simulink model "Refined_Model_43_Elec5_ch"  (R2020b)
settings: Solver=VariableStepAuto  StartTime=0.0  StopTime=16000  RelTol=1e-3
values from neighbouring files (symbols this model uses):
  Cx = VehicleDefine(7,3)    [BEV_Script_GPS.m]    (also in ICEBEV_Script_GPS.m; ICE_Script_GPS.m)
  Dist = [1:length(FMSP1)]    [BEV_Script_GPS.m]    (also in ICEBEV_Script_GPS.m; ICE_Script_GPS.m)
  DynRolRad = VehicleDefine(5,3)    [BEV_Script_GPS.m]    (also in ICEBEV_Script_GPS.m; ICE_Script_GPS.m)
  Fr = VehicleDefine(13,3)    [BEV_Script_GPS.m]    (also in ICEBEV_Script_GPS.m; ICE_Script_GPS.m)
  g = VehicleDefine(14,3)    [BEV_Script_GPS.m]    (also in ICEBEV_Script_GPS.m; ICE_Script_GPS.m)
  IntpSlope = round(IntpSlope,1)    [BEV_Script_GPS.m]    (also in ICEBEV_Script_GPS.m; ICE_Script_GPS.m)
  MaxAcc = 1    [BEV_Script_GPS.m]    (also in ICEBEV_Script_GPS.m; ICE_Script_GPS.m)
  MaxDec = 1    [BEV_Script_GPS.m]    (also in ICEBEV_Script_GPS.m; ICE_Script_GPS.m)
  MaxSpeedProfile = repelem(SegSPLatinmps,SegLeninm)    [BEV_Script_GPS.m]    (also in ICEBEV_Script_GPS.m; ICE_Script_GPS.m)
  Mtot = Mv+Me+Mt    [BEV_Script_GPS.m]    (also in ICEBEV_Script_GPS.m; ICE_Script_GPS.m)
  rho = VehicleDefine(6,3)    [BEV_Script_GPS.m]    (also in ICEBEV_Script_GPS.m; ICE_Script_GPS.m)
  s = divisors(length(MaxSpeedProfile))    [BEV_Script_GPS.m]    (also in ICEBEV_Script_GPS.m; ICE_Script_GPS.m; interparc.m = totalsplinelength*t)
  SegSPLatinmps = (sqrt(aMaxLat*g*CurRadinm))    [BEV_Script_GPS.m]    (also in ICEBEV_Script_GPS.m; ICE_Script_GPS.m)
  Stoptimes = readmatrix('GPS Routes and OC\Brno - Vienna - OC_description.xlsx','Sheet','Stop')    [BEV_Script_GPS.m]    (also in ICEBEV_Script_GPS.m = readmatrix('GPS Routes and OC\Turin - Lyon - OC_description.; ICE_Script_GPS.m = readmatrix('GPS Routes and OC\Dusseldorf - Cologne - OC_desc)
  Sx = VehicleDefine(8,3)    [BEV_Script_GPS.m]    (also in ICEBEV_Script_GPS.m; ICE_Script_GPS.m)
  W_mmax = VehicleDefine(26,3)    [BEV_Script_GPS.m]    (also in ICEBEV_Script_GPS.m = Etr(1,3))
undefined symbols (not defined in the file or in its folder): CovDist, G1Inprpm, Ion, Lithium, SegNo
libraries: fl_lib x8, nesl_utility x4, ee_lib x3, powerlib x2, electricdrivelib x1, sdl_lib x1, autolibshared x1
settings Model: Creator=Kshitij  LastModifiedBy=Kshitij
settings SolverCC: MaxConsecutiveMinStep=100000  ZeroCrossAlgorithm=Adaptive
settings DebuggingCC: IgnoredZcDiagnostic=none

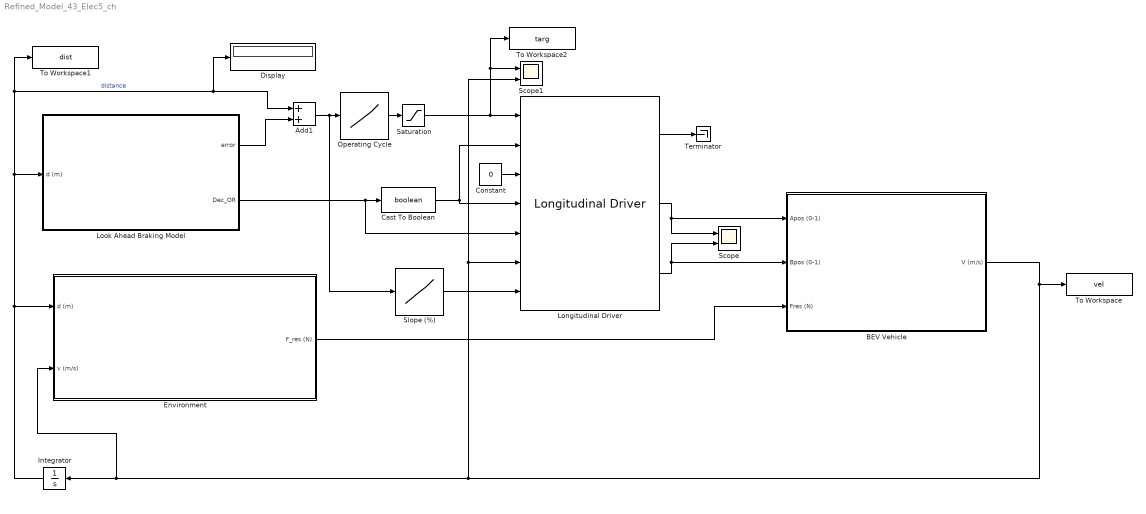
== system Refined_Model_43_Elec5_ch ==
  Add1 : Sum
  BEV Vehicle : Subsystem
  Cast To Boolean : DataTypeConversion  OutDataTypeStr=boolean
  Constant : Constant  Value=0
  Display : Display
  Environment : Subsystem
  Integrator : Integrator
  Longitudinal Driver : autolibshared/Longitudinal Driver  extAccelOvr=on  extDecelOvr=on  extAccelHld=off  extDecelHld=off  extAccelZero=off  extDecelZero=off  cntrlType=PI  shftType=None  velUnits=m/s  gearOut=off  Kp=200  Ki=150  Kff=0  Kg=0  VehVelVec=[0 100]  KffVec=[.1 .1]  KpVec=[10 10]  KiVec=[5 5]  KgVec=[0 0]  m=1500  Kpt=3000  tau=.1  L=2  aR=200  bR=2.5  cR=.5  g=9.81  vnom=100  Kaw=0  tauerr=0  tauPt=2  GearInit=0  tShift=.1  pdlVec=[0.1 0.4 0.5 0.9]  upShftTbl=[-1 12.9375 26.4375 39.9375 51.18749999999999 62.4375 72.84375 83.25;-1 16.3125 29.8125 43.3125 54.5624 65.8125 76.78125 87.75;-1 19.6875 33.1875 46.68749999999999 57.9375 69.1875 80.71875 92.25;-1 33 52.5 77.25 100.5 138.75 161.875 185]  dwnShftTbl=[1 9.5625 23.0625 36.5625 47.8125 59.0625 68.90625 78.75;1 12.9375 26.4375 39.9375 51.18749999999999 62.4375 72.84375 83.25;1 16.3125 29.8125 43.3125 54.562499 65.8125 76.78125 87.75;1 19.6875 33.1875 46.68749999999999 57.9375 69.1875 80.71875 92.25]  tClutch=.5  tRev=.5  tPark=120  aMode=1  UpGearVec="[0  1  2  3  4  5  6  7]"  DownGearVec="[1  2  3  4  5  6  7  8]"
      settings: SourceProductBaseCode=PW,DR,MT,UV,VE
  Look Ahead Braking Model : Subsystem
  Operating Cycle : Lookup_n-D  NumberOfTableDimensions=1  BreakpointsForDimension1=Dist  BreakpointsForDimension2=G1Inprpm  Table=MaxSpeedProfile  InterpMethod=Linear Lagrange  InternalRulePriority=Speed  RndMeth=Simplest  InputSameDT=on
  Saturation : Saturate  UpperLimit=inf  LowerLimit=0
  Scope : Scope  NumInputPorts=2
  Scope1 : Scope  NumInputPorts=2
  Slope (%) : Lookup_n-D  NumberOfTableDimensions=1  BreakpointsForDimension1=Dist  Table=IntpSlope  InternalRulePriority=Speed  RndMeth=Simplest  InputSameDT=on
  Terminator : Terminator
  To Workspace : ToWorkspace  VariableName=vel  SaveFormat=Timeseries  SampleTime=-1
  To Workspace1 : ToWorkspace  VariableName=dist  SaveFormat=Timeseries  SampleTime=-1
  To Workspace2 : ToWorkspace  VariableName=targ  SaveFormat=Timeseries  SampleTime=-1
  wires:
  Longitudinal Driver/2 -> Scope/1, BEV Vehicle/1(Apos (0-1))
  Integrator/1 -> To Workspace1/1, Add1/1, Display/1, Look Ahead Braking Model/1(d (m)), Environment/1(d (m))  "distance"
  Slope (%)/1 -> Longitudinal Driver/7
  Operating Cycle/1 -> Saturation/1
  Longitudinal Driver/1 -> Terminator/1
  Look Ahead Braking Model/2(Dec_OR) -> Longitudinal Driver/5, Cast To Boolean/1
  Cast To Boolean/1 -> Longitudinal Driver/4, Longitudinal Driver/2
  Add1/1 -> Slope (%)/1, Operating Cycle/1
  Look Ahead Braking Model/1(error) -> Add1/2
  BEV Vehicle/1(V (m/s)) -> To Workspace/1, Scope1/2, Longitudinal Driver/6, Environment/2(v (m/s)), Integrator/1
  Longitudinal Driver/3 -> BEV Vehicle/2(Bpos (0-1)), Scope/2
  Environment/1(F_res (N)) -> BEV Vehicle/3(Fres (N))
  Saturation/1 -> To Workspace2/1, Scope1/1, Longitudinal Driver/1
  Constant/1 -> Longitudinal Driver/3

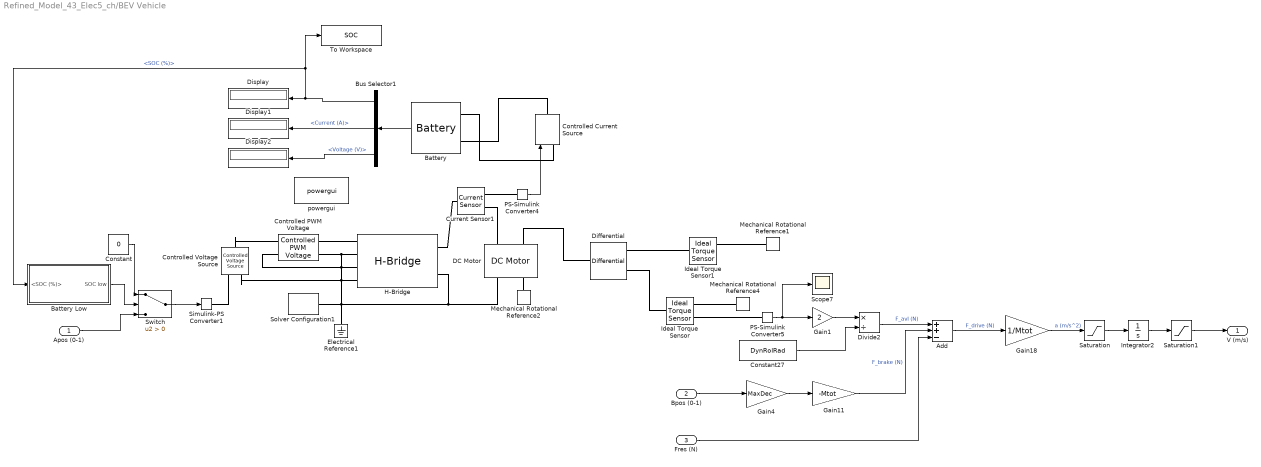
== system Refined_Model_43_Elec5_ch/BEV Vehicle ==
  Apos (0-1) : Inport
  Bpos (0-1) : Inport  Port=2
  Fres (N) : Inport  Port=3
  Add : Sum  Inputs=++-
  Battery : electricdrivelib/Extra Sources/Battery  BatType=Lithium-Ion  ShowTempParam=off  ThermalPreset=no  ShowAgeParam=off  NomV=V  NomQ=C_cap  SOC=100  Batt_Tr=15  PresetModel=on  MaxQ=470  MinV=562.5  FullV=872.9904  Dis_rate=204.3478  R=0.015957  Normal_OP=425.0435  expZone="[810.2894       23.0913]"  current=[6.5 13 32.5]  Units=Time  Tci=20  NomT=20  T2=-30  MaxQ2=4.8  FullV2=7.1  Normal_OP2=5.655  expZone2="[6.58           1]"  Rca=0.6  ti=2000  Dp=0  Neq0=0  Tsim=1e6  Ta1=25  Qeol=5.4*0.9  Reol=0.013333*1.2  Char_age=[2.3478, 3]  Dis_age=[2.3478, 10]  N1=1500  N2=10500  N3=1000  N4=1400  Ta2=45  N5=950
  Battery Low : Subsystem
  Bus Selector1 : BusSelector  OutputSignals=SOC (%),Current (A),Voltage (V)
  Constant : Constant  Value=0
  Constant27 : Constant  Value=DynRolRad
  Controlled Current Source : powerlib/Electrical Sources/Controlled Current Source  Initialize=on  Source_Type=DC  Amplitude=0  Phase=0  Frequency=0  Measurements=None
  Controlled PWM Voltage : ee_lib/Integrated Circuits/Controlled PWM Voltage  F=1000 Hz  TD=0 s  pulse_width_offset=0 s  pulse_min=0 s  Vmin=0 V  Vmax=2.5 V  Vm=V V  pwm_or_av=2  event_type=1  sample_time=1e-6 s  u_min=0  u_max=1
  Controlled Voltage Source : fl_lib/Electrical/Electrical Sources/Controlled Voltage Source
  Current Sensor1 : fl_lib/Electrical/Electrical Sensors/Current Sensor
  DC Motor : ee_lib/Electromechanical/Brushed Motors/DC Motor  field_option=ee.enum.field_option.pm  Rf=100 Ohm  Lf=1 H  Laf=0.15 H  If0=0 A  parameterization=ee.enum.dcparam_option.load_speed  Ra=3.9 Ohm  La=12e-6 H  emf_or_torque=ee.enum.emf_or_torque.kv  Kv=0.072e-3 V/rpm  Ki=6.876e-4 N*m/A  T_stall=0.24e-3 N*m  w_max=W_mmax rpm  w_rated=W_mmax-200 rpm  P_rated=P_mmax kW  V_rated=V V  J=0.01 g*cm^2  lam_param=ee.enum.lam_param.damping  lam=0 N*m/(rad/s)  i_noload=0 A  V_i_noload=1.5 V  speed0=0 rpm  enable_fault_armature=ee.enum.faults.faultEnable.no  rev_faulted=1 / 3  G_faulted_armature=1e-5 S  fault_trigger_armature=ee.enum.faults.faultTrigger.temporal  t_fault_armature=1 s  max_permissible_current_armature=inf A  t_fail_on_current_armature=1 s  enable_fault_field=ee.enum.faults.faultEnable.no  G_faulted_field=1e-5 S  fault_trigger_field=ee.enum.faults.faultTrigger.temporal  t_fault_field=1 s  max_permissible_current_field=inf A  t_fail_on_current_field=1 s  fault_action=ee.enum.faults.faultAction.none  alpha=3.93e-3 1/K  Tmeas=25 degC  thermal_mass=100 J/K  initial_temperature=25 degC
  Differential : sdl_lib/Gears/Differential  driveshaft_location=sdl.enum.differential_orientation.right  cd_ratio=FDR  friction_model=sdl.enum.gear_friction.none  mu_visc=[0, 0] N*m/(rad/s)  efficiency=[.85, .92]  temperature_TLU=[280, 300, 320] K  efficiency_ss_TLU=[.95, .9, .85]  efficiency_cd_TLU=[.95, .9, .85]  pwr_thr=[.001, .001] W  thermal_mass=50 J/K  T_init=300 K  model_inertia=simscape.enum.onoff.off  carrier_inertia=0.001 kg*m^2  planet_inertia=0.001 kg*m^2
      settings: SourceProductBaseCode=LD
  Display : Display
  Display1 : Display
  Display2 : Display
  Divide2 : Product  Inputs=*/
  Electrical Reference1 : fl_lib/Electrical/Electrical Elements/Electrical Reference
  Gain1 : Gain  Gain=2
  Gain11 : Gain  Gain=-Mtot
  Gain18 : Gain  Gain=1/Mtot
  Gain4 : Gain  Gain=MaxDec
  H-Bridge : ee_lib/Semiconductors & Converters/Converters/H-Bridge  supply_ports=ee.enum.supply_ports.hidesupply  Venable=2.5 V  Vmax=5.0 V  Vreverse=2.5 V  Vbrake=2.5 V  Vm=V V  pwm_or_av=ee.enum.pwm_or_av.averaged  regenerative_braking_mode=ee.enum.converters.regenerative_braking_mode.depends_on_rev  discontinuous=ee.enum.current_profile.continuous  freewheeling_mode=ee.enum.converters.freewheeling_mode.one_switch_one_diode  Ron=0.1 Ohm  Don=0.05 Ohm  Goff=1e-6 S  Rload=10 Ohm  Lload=1e-5 H  F=10 kHz  thermal_mass=100 J/K  initial_temperature=298.15 K  Ron2=0.1 Ohm  Don2=0.05 Ohm  Tmeas=298.15 K  Tmeas2=398.15 K
  Ideal Torque Sensor : fl_lib/Mechanical/Mechanical Sensors/Ideal Torque Sensor
  Ideal Torque Sensor1 : fl_lib/Mechanical/Mechanical Sensors/Ideal Torque Sensor
  Integrator2 : Integrator  ContinuousStateAttributes='acceleration'
  Mechanical Rotational Reference1 : fl_lib/Mechanical/Rotational Elements/Mechanical Rotational Reference
  Mechanical Rotational Reference2 : fl_lib/Mechanical/Rotational Elements/Mechanical Rotational Reference
  Mechanical Rotational Reference4 : fl_lib/Mechanical/Rotational Elements/Mechanical Rotational Reference
  PS-Simulink Converter4 : nesl_utility/PS-Simulink Converter  PhysicalDomain=network_engine_domain  SubClassName=ps_output  LeftPortType=input  RightPortType=output  PseudoPeriodic=off  Frequencies=[]  Unit=inherit  AffineConversion=off
      settings: SourceProductBaseCode=PW,SS
  PS-Simulink Converter5 : nesl_utility/PS-Simulink Converter  PhysicalDomain=network_engine_domain  SubClassName=ps_output  LeftPortType=input  RightPortType=output  PseudoPeriodic=off  Frequencies=[]  Unit=inherit  AffineConversion=off
      settings: SourceProductBaseCode=PW,SS
  Saturation : Saturate  UpperLimit=MaxAcc  LowerLimit=-(MaxDec)
  Saturation1 : Saturate  UpperLimit=inf  LowerLimit=0
  Scope7 : Scope
  Simulink-PS Converter1 : nesl_utility/Simulink-PS Converter  PhysicalDomain=network_engine_domain  SubClassName=ps_input  LeftPortType=input  RightPortType=output  PseudoPeriodic=off  Frequencies=[]  NoiseDistribution=none  NoiseParameters=[]  Unit=1  AffineConversion=off  FilteringAndDerivatives=provide  SimscapeFilterOrder=1  InputFilterTimeConstant=0.001  UdotUserProvided=0
      settings: SourceProductBaseCode=PW,SS
  Solver Configuration1 : nesl_utility/Solver Configuration  PhysicalDomain=network_engine_domain  SubClassName=solver  LeftPortType=input  RightPortType=generic  Tones=[]  Harmonics=[]  SimulateNoise=off  Profile=off  UseLocalSampling=off  EnableSwitchedLinearOptims=on  FrequencyDomain=off  UseCCode=off  RelTol=0.001  AbsTol=1e-06  MinStep=1e-09  ToWorkspace=off  RevertToSquareIcSolve=off  NumHomotopyIterations=100  PhasorMode=off  PhasorModeNumHarmonics=1  DoDC=off  ResidualTolerance=1e-09  UseLocalSolver=off  LocalSolverChoice=NE_BACKWARD_EULER_ADVANCER  LocalSolverSampleTime=0.001  DoFixedCost=off  MaxNonlinIter=3  MaxModeIter=2  ComputeImpulses=off  ImpulseIterations=2  LinearAlgebra=auto  EquationFormulation=NE_TIME_EF  DelaysMemoryBudget=1024  AutomaticFiltering=on  FilteringTimeConstant=0.001  PartitionStorageMethod=AS_NEEDED  PartitionMemoryBudget=1024  PartitionMethod=ROBUST
      settings: SourceProductBaseCode=PW,SS
  Switch : Switch  Criteria=u2 > Threshold
  To Workspace : ToWorkspace  VariableName=SOC  SaveFormat=Timeseries  SampleTime=-1
  powergui : powerlib/powergui  Priority=1  SimulationMode=Continuous  SampleTime=50e-6  frequency=60  Iterations=50  frequencyindice=0  Pbase=100e6  ErrMax=1e-4  UnitsV=kV  UnitsW=MW  buscounter=0  FunctionMessages=off  echomessages=off  EnableUseOfTLC=off  CurrentSourceSwitches=off  DisableSnubberDevices=off  DisableRonSwitches=off  DisableVfSwitches=off  DisplayEquations=off  AutomaticDiscreteSolvers=off  SolverType=Tustin/Backward Euler (TBE)  Interpol=off  ExternalGateDelay=off  methode=off  Ts=100  x0status=blocks  SPID=on  SwTol=0  HookPort=off  NonlinearTolerance=1e-4  nMaxIteration=100  ContinueOnMaxIteration=off  RestoreLinks=warning  ResistiveCurrentMeasurement=off  Frange=[0:2:500]  Ylog=off  Xlog=on  ShowGrid=off  save=off  variable=ZData  structure=0  ZoomFFT=off  StartTime=0.0  cycles=1  DisplayStyle=1  fundamental=60  FreqAxis=off  MaxFrequency=1000  frequencyindicesteady=1  RmsSteady=1  display=off
  V (m/s) : Outport
  wires:
  PS-Simulink Converter4/1 -> Controlled Current Source/1
  Constant27/1 -> Divide2/2
  Add/1 -> Gain18/1  "F_drive (N)"
  Fres (N)/1 -> Add/3
  Bpos (0-1)/1 -> Gain4/1
  Integrator2/1 -> Saturation1/1
  Bus Selector1/1 -> To Workspace/1, Battery Low/1(<SOC (%)>), Display/1  "<SOC (%)>"
  PS-Simulink Converter5/1 -> Gain1/1, Scope7/1
  Bus Selector1/3 -> Display2/1  "<Voltage (V)>"
  Bus Selector1/2 -> Display1/1  "<Current (A)>"
  Gain11/1 -> Add/2  "F_brake (N)"
  Gain4/1 -> Gain11/1
  Gain1/1 -> Divide2/1
  Divide2/1 -> Add/1  "F_avl (N)"
  Gain18/1 -> Saturation/1  "a (m/s^2)"
  Battery/1 -> Bus Selector1/1
  Saturation/1 -> Integrator2/1
  Saturation1/1 -> V (m/s)/1
  Apos (0-1)/1 -> Switch/3
  Switch/1 -> Simulink-PS Converter1/1
  Battery Low/1(SOC low) -> Switch/2
  Constant/1 -> Switch/1
  connections:
  Solver Configuration1/RConn1 -- Electrical Reference1/LConn1 -- DC Motor/RConn1 -- H-Bridge/RConn2 -- H-Bridge/LConn4 -- Controlled Voltage Source/RConn2 -- H-Bridge/LConn3 -- H-Bridge/LConn2 -- Controlled PWM Voltage/RConn2 -- Controlled PWM Voltage/LConn2
  Controlled Current Source/LConn1 -- Battery/LConn1
  Differential/LConn1 -- DC Motor/LConn2
  Current Sensor1/RConn2 -- DC Motor/LConn1
  PS-Simulink Converter4/LConn1 -- Current Sensor1/RConn1
  Controlled Voltage Source/LConn1 -- Controlled PWM Voltage/LConn1
  Controlled PWM Voltage/RConn1 -- H-Bridge/LConn1
  Ideal Torque Sensor1/LConn1 -- Differential/RConn2
  Simulink-PS Converter1/RConn1 -- Controlled Voltage Source/RConn1
  Mechanical Rotational Reference2/LConn1 -- DC Motor/RConn2
  H-Bridge/RConn1 -- Current Sensor1/LConn1
  Ideal Torque Sensor/LConn1 -- Differential/RConn1
  Battery/LConn2 -- Controlled Current Source/RConn1
  Mechanical Rotational Reference4/LConn1 -- Ideal Torque Sensor/RConn1
  Mechanical Rotational Reference1/LConn1 -- Ideal Torque Sensor1/RConn1
  PS-Simulink Converter5/LConn1 -- Ideal Torque Sensor/RConn2

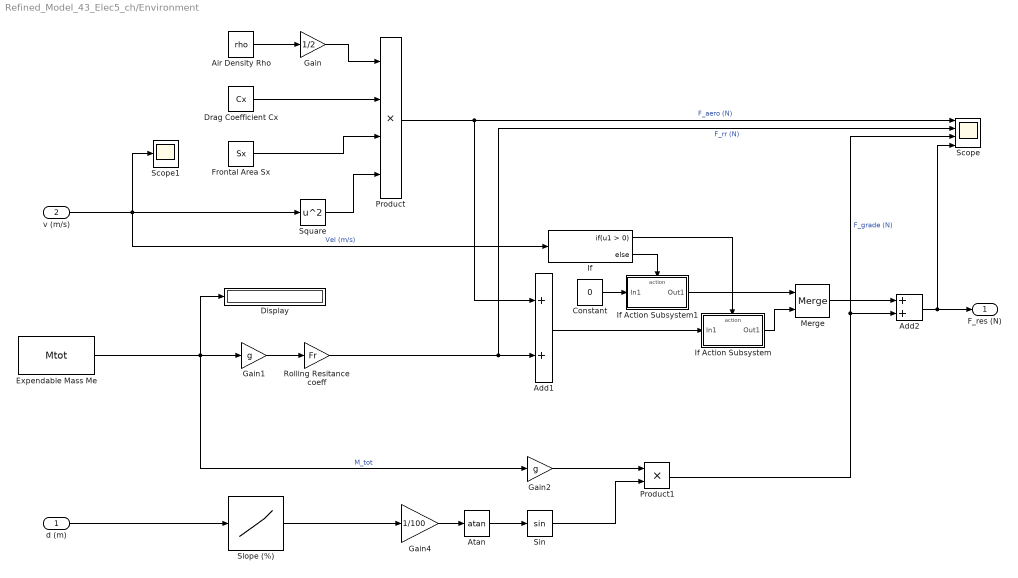
== system Refined_Model_43_Elec5_ch/Environment ==
  d (m) : Inport
  v (m/s) : Inport  Port=2
  Add1 : Sum
  Add2 : Sum
  Air Density Rho : Constant  Value=rho
  Atan : Trigonometry  Operator=atan
  Constant : Constant  Value=0
  Display : Display
  Drag Coefficient Cx : Constant  Value=Cx
  Expendable Mass Me : Constant  Value=Mtot
  Frontal Area Sx : Constant  Value=Sx
  Gain : Gain  Gain=1/2
  Gain1 : Gain  Gain=g
  Gain2 : Gain  Gain=g
  Gain4 : Gain  Gain=1/100
  If : If
  If Action Subsystem : Subsystem  TreatAsAtomicUnit=on
  If Action Subsystem1 : Subsystem  TreatAsAtomicUnit=on
  Merge : Merge
  Product : Product  Inputs=4
  Product1 : Product
  Rolling Resitance coeff : Gain  Gain=Fr
  Scope : Scope  NumInputPorts=4
  Scope1 : Scope
  Sin : Trigonometry
  Slope (%) : Lookup_n-D  NumberOfTableDimensions=1  BreakpointsForDimension1=Dist  Table=IntpSlope  InternalRulePriority=Speed  RndMeth=Simplest  InputSameDT=on
  Square : Math  Operator=square  SaturateOnIntegerOverflow=on
  F_res (N) : Outport
  wires:
  Expendable Mass Me/1 -> Gain2/1, Display/1, Gain1/1  "M_tot"
  Gain/1 -> Product/1
  Sin/1 -> Product1/2
  Product1/1 -> Scope/3, Add2/2  "F_grade (N)"
  Air Density Rho/1 -> Gain/1
  Drag Coefficient Cx/1 -> Product/2
  v (m/s)/1 -> Scope1/1, Square/1, If/1  "Vel (m/s)"
  d (m)/1 -> Slope (%)/1
  Gain2/1 -> Product1/1
  Rolling Resitance coeff/1 -> Scope/2, Add1/2  "F_rr (N)"
  Square/1 -> Product/4
  Gain1/1 -> Rolling Resitance coeff/1
  Product/1 -> Scope/1, Add1/1  "F_aero (N)"
  Frontal Area Sx/1 -> Product/3
  If/1 -> If Action Subsystem/Action
  If/2 -> If Action Subsystem1/Action
  If Action Subsystem1/1(Out1) -> Merge/1
  Add1/1 -> If Action Subsystem/1(In1)
  If Action Subsystem/1(Out1) -> Merge/2
  Constant/1 -> If Action Subsystem1/1(In1)
  Merge/1 -> Add2/1
  Add2/1 -> F_res (N)/1, Scope/4
  Slope (%)/1 -> Gain4/1
  Atan/1 -> Sin/1
  Gain4/1 -> Atan/1

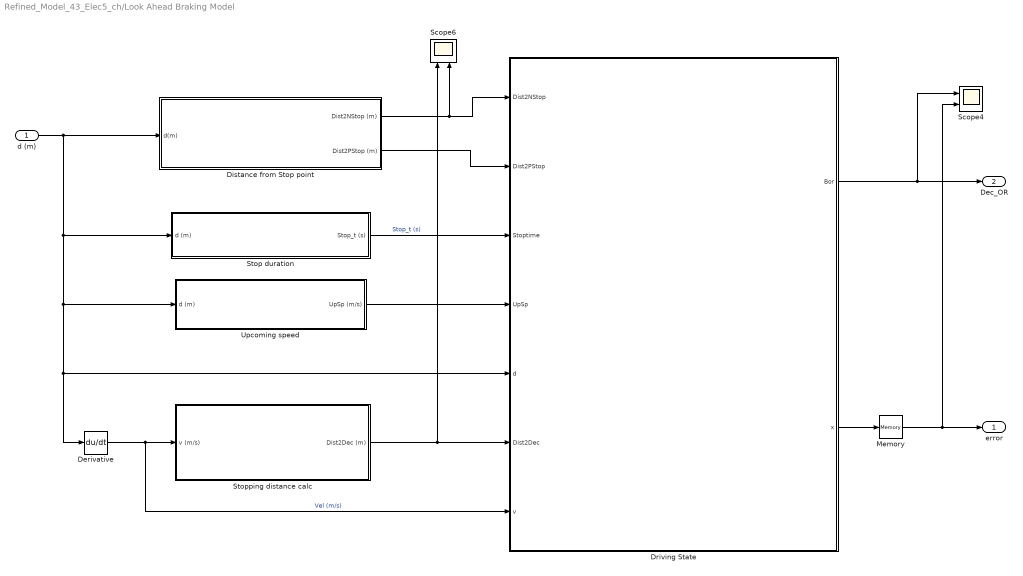
== system Refined_Model_43_Elec5_ch/Look Ahead Braking Model ==
  d (m) : Inport
  Derivative : Derivative
  Distance from Stop point : Subsystem
  Driving State : Stateflow chart  TreatAsAtomicUnit=on
      settings: PortSchema="{\"entries\":[{\"content\":{\"sides\":[{\"content\":{\"connectorIds\":[\"In2\",\"In3\",\"In4\",\"In5\",\"In6\",\"In1\",\"In7\"]},\"type\":\"ConnectorPlacement.EquallySpacedRectSide\",\"uuid\":\"d2ffa8ce-717b-462a-89f0-d2e290a1049a\"},{\"content\":{\"connectorIds\":[\"Out1\",\"Out2\"],\"side\":\"RIGHT\"},\"type\":\"ConnectorPlacement.EquallySpacedRectSide\",\"uuid\":\"23dd838e-bde8-43eb-b85c-28483cc72b3d\"},{\"content\":{\"connectorIds\":[],\"side\":\"TOP\"},\"type\":\"ConnectorPlacement.EquallySpacedRectSide\",\"uuid\":\"db6c289e-ad0a-41c0-bd77-f5e27867e32c\"},{\"content\":{\"connectorIds\":[],\"side\":\"HIDDEN\"},\"type\":\"ConnectorPlacement.EquallySpacedRectSide\",\"uuid\":\"2289313c-09ae-4c3c-923e-5092cac5b78d\"}]},\"type\":\"ConnectorPlacement.EquallySpacedConnector\",\"uuid\":\"13f19205-7a9b-4362-9535-522c20ce3cd1\"}],\"packageUris\":[\"http://schema.mathworks.com/mf0/Connector/R2020b\"],\"version\":\"1.0\"}"
  Memory : Memory
  Scope4 : Scope  NumInputPorts=2
  Scope6 : Scope  NumInputPorts=2
  Stop duration : Subsystem
  Stopping distance calc : Subsystem
  Upcoming speed : Subsystem
  error : Outport
  Dec_OR : Outport  Port=2
  wires:
  Derivative/1 -> Driving State/7(v), Stopping distance calc/1(v (m/s))  "Vel (m/s)"
  Distance from Stop point/1(Dist2NStop (m)) -> Scope6/2, Driving State/2(Dist2NStop)
  Distance from Stop point/2(Dist2PStop (m)) -> Driving State/3(Dist2PStop)
  Stop duration/1(Stop_t (s)) -> Driving State/4(Stoptime)  "Stop_t (s)"
  Stopping distance calc/1(Dist2Dec (m)) -> Scope6/1, Driving State/1(Dist2Dec)
  Upcoming speed/1(UpSp (m/s)) -> Driving State/5(UpSp)
  Driving State/2(x) -> Memory/1
  Driving State/1(Bor) -> Scope4/1, Dec_OR/1
  d (m)/1 -> Derivative/1, Driving State/6(d), Upcoming speed/1(d (m)), Stop duration/1(d (m)), Distance from Stop point/1(d(m))
  Memory/1 -> Scope4/2, error/1

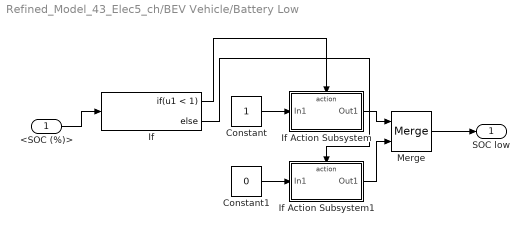
== system Refined_Model_43_Elec5_ch/BEV Vehicle/Battery Low ==
  <SOC (%)> : Inport
  Constant : Constant
  Constant1 : Constant  Value=0
  If : If  IfExpression=u1 < 1
  If Action Subsystem : Subsystem  TreatAsAtomicUnit=on
  If Action Subsystem1 : Subsystem  TreatAsAtomicUnit=on
  Merge : Merge
  SOC low : Outport
  wires:
  If/1 -> If Action Subsystem/Action
  Constant1/1 -> If Action Subsystem1/1(In1)
  If/2 -> If Action Subsystem1/Action
  If Action Subsystem/1(Out1) -> Merge/1
  If Action Subsystem1/1(Out1) -> Merge/2
  Constant/1 -> If Action Subsystem/1(In1)
  Merge/1 -> SOC low/1
  <SOC (%)>/1 -> If/1

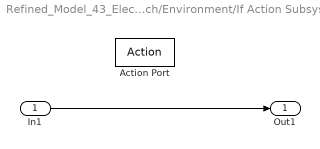
== system Refined_Model_43_Elec5_ch/Environment/If Action Subsystem ==
  In1 : Inport
  Action Port : ActionPort  ActionPortLabel=if(u1 > 0)
  Out1 : Outport
  wires:
  In1/1 -> Out1/1

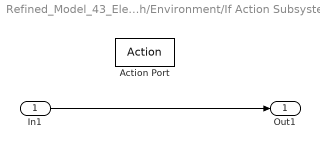
== system Refined_Model_43_Elec5_ch/Environment/If Action Subsystem1 ==
  In1 : Inport
  Action Port : ActionPort  ActionPortLabel=else
  Out1 : Outport
  wires:
  In1/1 -> Out1/1

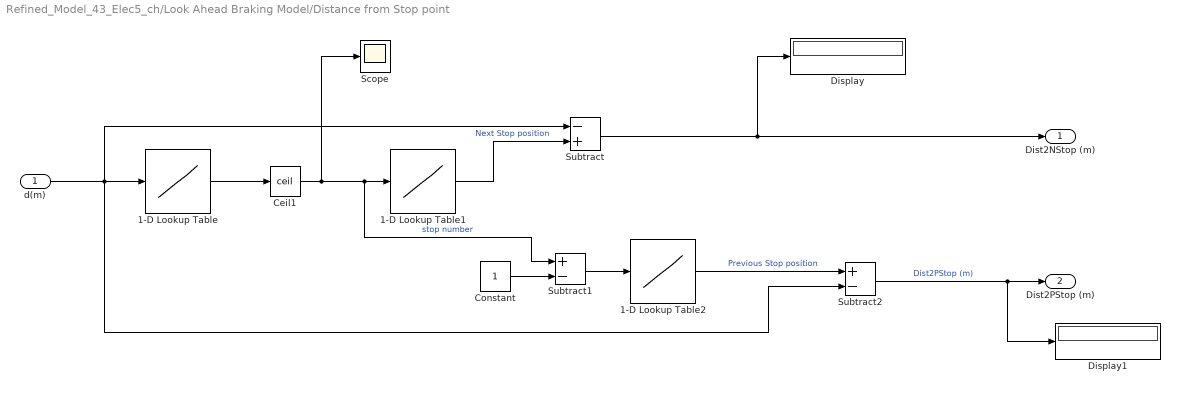
== system Refined_Model_43_Elec5_ch/Look Ahead Braking Model/Distance from Stop point ==
  d(m) : Inport
  1-D Lookup Table : Lookup_n-D  NumberOfTableDimensions=1  BreakpointsForDimension1=Stoptimes(:,1)  Table=1:length(Stoptimes(:,1))  InternalRulePriority=Speed  RndMeth=Simplest  InputSameDT=on
  1-D Lookup Table1 : Lookup_n-D  NumberOfTableDimensions=1  BreakpointsForDimension1=1:length(Stoptimes(:,1))  Table=Stoptimes(:,1)  InternalRulePriority=Speed  RndMeth=Simplest  InputSameDT=on
  1-D Lookup Table2 : Lookup_n-D  NumberOfTableDimensions=1  BreakpointsForDimension1=1:length(Stoptimes(:,1))  Table=Stoptimes(:,1)  InternalRulePriority=Speed  RndMeth=Simplest  InputSameDT=on
  Ceil1 : Rounding  Operator=ceil
  Constant : Constant
  Display : Display
  Display1 : Display
  Scope : Scope
  Subtract : Sum  Inputs=-+
  Subtract1 : Sum  Inputs=+-
  Subtract2 : Sum  Inputs=+-
  Dist2NStop (m) : Outport
  Dist2PStop (m) : Outport  Port=2
  wires:
  1-D Lookup Table2/1 -> Subtract2/1  "Previous Stop position"
  Ceil1/1 -> Scope/1, Subtract1/1, 1-D Lookup Table1/1  "stop number"
  d(m)/1 -> Subtract2/2, Subtract/1, 1-D Lookup Table/1
  Constant/1 -> Subtract1/2
  Subtract1/1 -> 1-D Lookup Table2/1
  1-D Lookup Table/1 -> Ceil1/1
  1-D Lookup Table1/1 -> Subtract/2  "Next Stop position"
  Subtract2/1 -> Display1/1, Dist2PStop (m)/1  "Dist2PStop (m)"
  Subtract/1 -> Display/1, Dist2NStop (m)/1

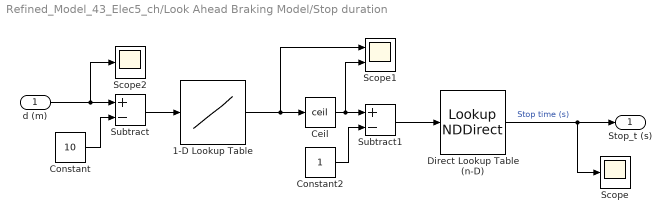
== system Refined_Model_43_Elec5_ch/Look Ahead Braking Model/Stop duration ==
  d (m) : Inport
  1-D Lookup Table : Lookup_n-D  NumberOfTableDimensions=1  BreakpointsForDimension1=Stoptimes(:,1)  Table=1:length(Stoptimes(:,1))  InternalRulePriority=Speed  RndMeth=Simplest  InputSameDT=on
  Ceil : Rounding  Operator=ceil
  Constant : Constant  Value=10
  Constant2 : Constant
  Direct Lookup Table (n-D) : LookupNDDirect  NumberOfTableDimensions=1  Table=Stoptimes(:,2)
  Scope : Scope
  Scope1 : Scope  NumInputPorts=2
  Scope2 : Scope
  Subtract : Sum  Inputs=+-
  Subtract1 : Sum  Inputs=+-
  Stop_t (s) : Outport
  wires:
  1-D Lookup Table/1 -> Scope1/1, Ceil/1
  d (m)/1 -> Subtract/1, Scope2/1
  Subtract1/1 -> Direct Lookup Table (n-D)/1
  Direct Lookup Table (n-D)/1 -> Stop_t (s)/1, Scope/1  "Stop time (s)"
  Ceil/1 -> Scope1/2, Subtract1/1
  Constant2/1 -> Subtract1/2
  Subtract/1 -> 1-D Lookup Table/1
  Constant/1 -> Subtract/2

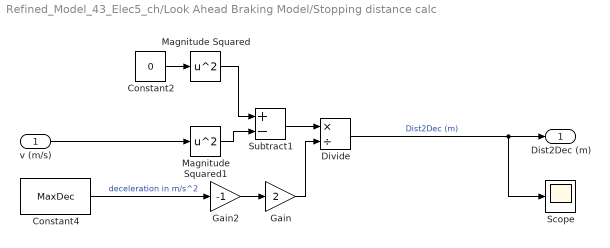
== system Refined_Model_43_Elec5_ch/Look Ahead Braking Model/Stopping distance calc ==
  v (m/s) : Inport
  Constant2 : Constant  Value=0
  Constant4 : Constant  Value=MaxDec
  Divide : Product  Inputs=*/
  Gain : Gain  Gain=2
  Gain2 : Gain  Gain=-1
  Magnitude Squared : Math  Operator=square  SaturateOnIntegerOverflow=on
  Magnitude Squared1 : Math  Operator=square  SaturateOnIntegerOverflow=on
  Scope : Scope
  Subtract1 : Sum  Inputs=+-
  Dist2Dec (m) : Outport
  wires:
  Divide/1 -> Dist2Dec (m)/1, Scope/1  "Dist2Dec (m)"
  Subtract1/1 -> Divide/1
  Magnitude Squared1/1 -> Subtract1/2
  Constant4/1 -> Gain2/1  "deceleration in m/s^2"
  Magnitude Squared/1 -> Subtract1/1
  Gain/1 -> Divide/2
  Gain2/1 -> Gain/1
  Constant2/1 -> Magnitude Squared/1
  v (m/s)/1 -> Magnitude Squared1/1

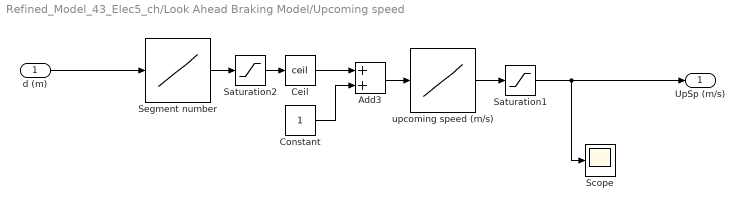
== system Refined_Model_43_Elec5_ch/Look Ahead Braking Model/Upcoming speed ==
  d (m) : Inport
  Add3 : Sum
  Ceil : Rounding  Operator=ceil
  Constant : Constant
  Saturation1 : Saturate  UpperLimit=inf  LowerLimit=0
  Saturation2 : Saturate  UpperLimit=inf  LowerLimit=0
  Scope : Scope
  Segment number : Lookup_n-D  NumberOfTableDimensions=1  BreakpointsForDimension1=CovDist  BreakpointsForDimension2=G1Inprpm  Table=SegNo  InterpMethod=Linear Lagrange  InternalRulePriority=Speed  RndMeth=Simplest  InputSameDT=on
  upcoming speed (m/s) : Lookup_n-D  NumberOfTableDimensions=1  BreakpointsForDimension1=SegNo  BreakpointsForDimension2=G1Inprpm  Table=SegSPLatinmps  InterpMethod=Linear Lagrange  InternalRulePriority=Speed  RndMeth=Simplest  InputSameDT=on
  UpSp (m/s) : Outport
  wires:
  upcoming speed (m/s)/1 -> Saturation1/1
  Ceil/1 -> Add3/1
  Constant/1 -> Add3/2
  Add3/1 -> upcoming speed (m/s)/1
  d (m)/1 -> Segment number/1
  Saturation1/1 -> Scope/1, UpSp (m/s)/1
  Segment number/1 -> Saturation2/1
  Saturation2/1 -> Ceil/1

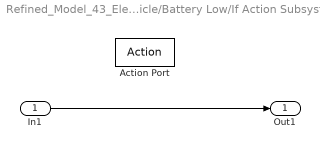
== system Refined_Model_43_Elec5_ch/BEV Vehicle/Battery Low/If Action Subsystem ==
  In1 : Inport
  Action Port : ActionPort  ActionPortLabel=if(u1 < 1)
  Out1 : Outport
  wires:
  In1/1 -> Out1/1

== system Refined_Model_43_Elec5_ch/BEV Vehicle/Battery Low/If Action Subsystem1 ==
  In1 : Inport
  Action Port : ActionPort  ActionPortLabel=else
  Out1 : Outport
  wires:
  In1/1 -> Out1/1

== stateflow chart Refined_Model_43_Elec5_ch/Look Ahead Braking Model/Driving State ==
  state Driving
    Bor = 0;
    error = x;
  state Stopping
    Bor = 1;
    error = x;
  state Calibration_pos
    Bor = 1;
    x = Dist2NStop;
  state Stopped
    Bor = 1;
    error = x;
  state Calibration_neg
    Bor = 1;
    x = Dist2PStop;
  (default) -> Driving : {x = 0;}
  Driving -> Stopping : [Dist2NStop <= Dist2Dec && UpSp <= 1]{Bor = 0;}
  Stopping -> Calibration_neg [order 1] : after(1,sec)[v == 0 && d > 0 && Dist2PStop <= 25 && Dist2Dec <= 0]{Bor = 1;}
  Stopping -> Calibration_pos [order 2] : after(1,sec)[v == 0 && d > 0 && Dist2NStop <= 25 && Dist2Dec == 0]{Bor = 1;}
  Stopped -> Driving : after((Stoptime/3.7)-1,sec)
  Calibration_pos -> Stopped : [v == 0]{x = x + Dist2NStop}
  Calibration_neg -> Stopped : [v == 0 ]{x = x - Dist2PStop}
  data: Bor output; Dist2Dec input; error local; Dist2NStop input; Dist2PStop input; Stoptime input; UpSp input; d input; v input; x output
